simulink model "ex2_C2"  (R2021a)
settings: Solver=VariableStepAuto  StartTime=0.0  StopTime=10.0  RelTol=1e-3
libraries: simulink x1
settings Model: Creator=Admin  LastModifiedBy=Admin

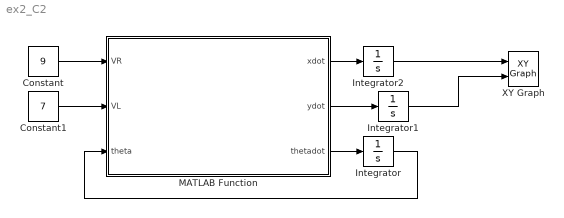
== system ex2_C2 ==
  Constant : Constant  Value=9
  Constant1 : Constant  Value=7
  Integrator : Integrator
  Integrator1 : Integrator
  Integrator2 : Integrator
  MATLAB Function : MATLAB Function  TreatAsAtomicUnit=on
  XY Graph : simulink/Sinks/XY Graph  xmin=-1  xmax=1  ymin=-1  ymax=1  st=-1
  wires:
  MATLAB Function/3(thetadot) -> Integrator/1
  Integrator/1 -> MATLAB Function/3(theta)
  MATLAB Function/1(xdot) -> Integrator2/1
  MATLAB Function/2(ydot) -> Integrator1/1
  Integrator2/1 -> XY Graph/1
  Integrator1/1 -> XY Graph/2
  Constant/1 -> MATLAB Function/1(VR)
  Constant1/1 -> MATLAB Function/2(VL)

== matlab function ex2_C2/MATLAB Function ==
  data: VR input; xdot output; VL input; theta input; ydot output; thetadot output
function [xdot, ydot, thetadot ]= fcn(VR,VL,theta)
d = 0.5;
xdot = ( VR+VL)/2*cos(theta);
ydot = (VR+VL)/2*sin(theta);
thetadot = (VR-VL)/d;
